simulink model "I_for_8_coils_diagonal_motion"  (R2021b)
settings: Solver=FixedStepAuto  StartTime=4400e-6  StopTime=14760e-6  FixedStep=50e-6  RelTol=1e-3
libraries: simulink x12
(part 1 of 6)
settings Model: Creator=teja  LastModifiedBy=teja

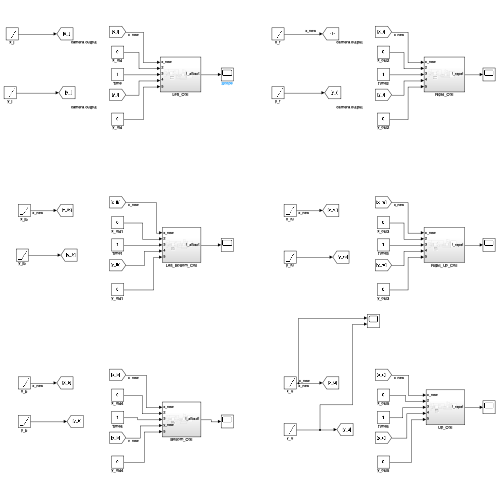
[thumbnail: Simulink's stored preview of the top-level diagram]
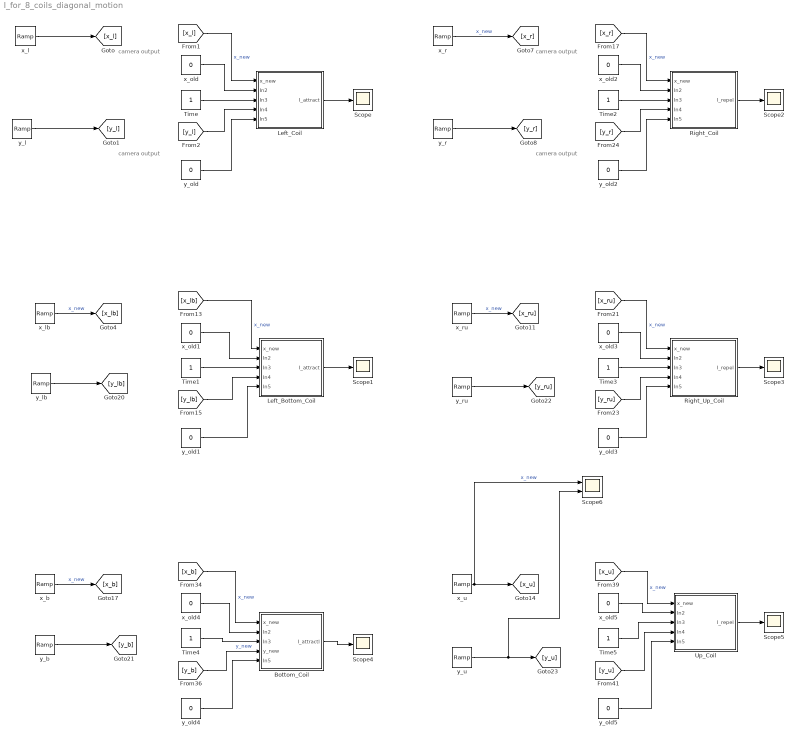
== system I_for_8_coils_diagonal_motion ==
  note: camera output
  note: camera output
  note: camera output
  note: camera output
  Bottom_Coil : Subsystem
  Left_Bottom_Coil : Subsystem
  Left_Coil : Subsystem
  Right_Coil : Subsystem
  Right_Up_Coil : Subsystem
  Scope{,1..5} (6 alike) : Scope
  Scope6 : Scope  NumInputPorts=2
  Time{,1..5} (6 alike) : Constant
  Up_Coil : Subsystem
  x_b : simulink/Sources/Ramp  slope=1  start=0  InitialOutput=-4400e-6
  x_l : simulink/Sources/Ramp  slope=1  start=0  InitialOutput=0
  x_lb : simulink/Sources/Ramp  slope=1  start=0  InitialOutput=0
  x_old{,1..5} (6 alike) : Constant  Value=0
  x_r : simulink/Sources/Ramp  slope=-1  start=0  InitialOutput=-4400e-6
  x_ru : simulink/Sources/Ramp  slope=-1  start=0  InitialOutput=0
  x_u : simulink/Sources/Ramp  slope=-1  start=0  InitialOutput=8800e-6
  y_b : simulink/Sources/Ramp  slope=1  start=0  InitialOutput=0
  y_l : simulink/Sources/Ramp  slope=1  start=0  InitialOutput=-8800e-6
  y_lb : simulink/Sources/Ramp  slope=1  start=0  InitialOutput=0
  y_old{,1..5} (6 alike) : Constant  Value=0
  y_r : simulink/Sources/Ramp  slope=-1  start=4400e-6  InitialOutput=0
  y_ru : simulink/Sources/Ramp  slope=-1  start=0  InitialOutput=0
  y_u : simulink/Sources/Ramp  slope=-1  start=0  InitialOutput=0
  wires:
  y_l/1 -> [y_l]
  x_lb/1 -> [x_lb]  "x_new"
  x_l/1 -> [x_l]
  y_lb/1 -> [y_lb]
  [x_l] -> Left_Coil/1(x_new)  "x_new"
  x_old/1 -> Left_Coil/2(In2)
  Time/1 -> Left_Coil/3(In3)
  [y_l] -> Left_Coil/4(In4)
  y_old/1 -> Left_Coil/5(In5)
  Left_Coil/1(I_attract) -> Scope/1
  [x_lb] -> Left_Bottom_Coil/1(x_new)  "x_new"
  x_old1/1 -> Left_Bottom_Coil/2(In2)
  Time1/1 -> Left_Bottom_Coil/3(In3)
  [y_lb] -> Left_Bottom_Coil/4(In4)
  y_old1/1 -> Left_Bottom_Coil/5(In5)
  Left_Bottom_Coil/1(I_attract) -> Scope1/1
  [x_b] -> Bottom_Coil/1(x_new)  "x_new"
  x_old4/1 -> Bottom_Coil/2(In2)
  Time4/1 -> Bottom_Coil/3(In3)
  [y_b] -> Bottom_Coil/4(y_new)  "y_new"
  y_old4/1 -> Bottom_Coil/5(In5)
  Bottom_Coil/1(I_attractl) -> Scope4/1
  [x_r] -> Right_Coil/1(x_new)  "x_new"
  x_old2/1 -> Right_Coil/2(In2)
  Time2/1 -> Right_Coil/3(In3)
  [y_r] -> Right_Coil/4(In4)
  y_old2/1 -> Right_Coil/5(In5)
  Right_Coil/1(I_repel) -> Scope2/1
  [x_ru] -> Right_Up_Coil/1(x_new)  "x_new"
  x_old3/1 -> Right_Up_Coil/2(In2)
  Time3/1 -> Right_Up_Coil/3(In3)
  [y_ru] -> Right_Up_Coil/4(In4)
  y_old3/1 -> Right_Up_Coil/5(In5)
  Right_Up_Coil/1(I_repel) -> Scope3/1
  [x_u] -> Up_Coil/1(x_new)  "x_new"
  x_old5/1 -> Up_Coil/2(In2)
  Time5/1 -> Up_Coil/3(In3)
  [y_u] -> Up_Coil/4(In4)
  y_old5/1 -> Up_Coil/5(In5)
  Up_Coil/1(I_repel) -> Scope5/1
  y_b/1 -> [y_b]
  x_b/1 -> [x_b]  "x_new"
  x_r/1 -> [x_r]  "x_new"
  y_r/1 -> [y_r]
  y_ru/1 -> [y_ru]
  x_ru/1 -> [x_ru]  "x_new"
  y_u/1 -> Scope6/2, [y_u]
  x_u/1 -> Scope6/1, [x_u]  "x_new"

== system I_for_8_coils_diagonal_motion/Bottom_Coil ==
  note: Inside coil, it is repulsive force, hence outside coil it generates attractive force
      |
      | Hence F increasing from -14 to -4
  note: Bot coming to this coil
  x_new : Inport
  In2 : Inport  Port=2
  In3 : Inport  Port=3
  y_new : Inport  Port=4
  In5 : Inport  Port=5
  Force_repel2 : Subsystem
  Left_Coil2 : Subsystem
  Required Current in Coil4 : MATLAB Function  TreatAsAtomicUnit=on
  z_new4 : Constant  Value=150e-6
  I_attractl : Outport
  wires:
  In2/1 -> Force_repel2/2(In2)
  In3/1 -> Force_repel2/3(In3)
  In5/1 -> Force_repel2/5(In5)
  x_new/1 -> Left_Coil2/1(x_new), Required Current in Coil4/7(x_new), Force_repel2/1(In1)
  Required Current in Coil4/1(I) -> I_attractl/1  "I_attract"
  Left_Coil2/4(Out4) -> Required Current in Coil4/6(dyn_dz)  "dyn/dz"
  y_new/1 -> Left_Coil2/2(y_new), Required Current in Coil4/8(y_new), Force_repel2/4(In4)
  Force_repel2/1(F_mag_x) -> [F_mag_xb]  "F_mag_x"
  z_new4/1 -> Left_Coil2/3(z_new)
  [F_mag_xb] -> Required Current in Coil4/1(F_xz_1)  "F_x"
  [F_mag_yb] -> Required Current in Coil4/2(F_yz_1)  "F_y"
  Force_repel2/2(F_mag_y) -> [F_mag_yb]
  Left_Coil2/2(Out2) -> Required Current in Coil4/4(dxn_dz)  "dxn/dz"
  Left_Coil2/1(Out1) -> Required Current in Coil4/3(dxp_dz)  "dxp/dz"
  Left_Coil2/3(Out3) -> Required Current in Coil4/5(dyp_dz)  "dyp/dz"

== system I_for_8_coils_diagonal_motion/Left_Bottom_Coil ==
  note: Inside coil, it is repulsive force, hence outside coil it generates attractive force
      |
      | Hence F increasing from -14 to -4
  note: Bot coming to this coil
  x_new : Inport
  In2 : Inport  Port=2
  In3 : Inport  Port=3
  In4 : Inport  Port=4
  In5 : Inport  Port=5
  Force_repel : Subsystem
  Left_Coil : Subsystem
  Required Current in Coil1 : MATLAB Function  TreatAsAtomicUnit=on
  z_new1 : Constant  Value=150e-6
  I_attract : Outport
  wires:
  In3/1 -> Force_repel/3(In3)
  In2/1 -> Force_repel/2(In2)
  x_new/1 -> Required Current in Coil1/7(x_new), Left_Coil/1(x_new), Force_repel/1(In1)
  [F_mag_ylb] -> Required Current in Coil1/2(F_yz_1)  "F_y"
  Force_repel/2(F_mag_y) -> [F_mag_ylb]
  Left_Coil/4(Out4) -> Required Current in Coil1/6(dyn_dz)  "dyn/dz"
  Force_repel/1(F_mag_x) -> [F_mag_xlb]  "F_mag_x"
  In5/1 -> Force_repel/5(In5)
  Required Current in Coil1/1(I) -> I_attract/1  "I_attract"
  [F_mag_xlb] -> Required Current in Coil1/1(F_xz_1)  "F_x"
  Left_Coil/1(Out1) -> Required Current in Coil1/3(dxp_dz)  "dxp/dz"
  In4/1 -> Required Current in Coil1/8(y_new), Left_Coil/2(y_new), Force_repel/4(In4)
  z_new1/1 -> Left_Coil/3(z_new)
  Left_Coil/2(Out2) -> Required Current in Coil1/4(dxn_dz)  "dxn/dz"
  Left_Coil/3(Out3) -> Required Current in Coil1/5(dyp_dz)  "dyp/dz"

== system I_for_8_coils_diagonal_motion/Left_Coil ==
  note: Inside coil, it is attractive force, hence outside coil it generates repulsive force
      |
      | Hence F increasing from 4 to 14
  x_new : Inport
  In2 : Inport  Port=2
  In3 : Inport  Port=3
  In4 : Inport  Port=4
  In5 : Inport  Port=5
  Force_attract : Subsystem
  Required Current in Coil : MATLAB Function  TreatAsAtomicUnit=on
  Right_Coil : Subsystem
  z_new : Constant  Value=150e-6
  I_attract : Outport
  wires:
  In2/1 -> Force_attract/2(In2)
  Required Current in Coil/1(I) -> I_attract/1  "I_attract"
  In4/1 -> Right_Coil/2(y_new), Required Current in Coil/8(y_new), Force_attract/4(In4)
  x_new/1 -> Right_Coil/1(x_new), Required Current in Coil/7(x_new), Force_attract/1(In1)
  In3/1 -> Force_attract/3(In3)
  Force_attract/2(F_mag_y) -> [F_mag_yl]
  Right_Coil/1(Out1) -> Required Current in Coil/3(dxp_dz)  "dxp/dz"
  In5/1 -> Force_attract/5(In5)
  z_new/1 -> Right_Coil/3(z_new)
  Right_Coil/2(Out2) -> Required Current in Coil/4(dxn_dz)  "dxn/dz"
  [F_mag_xl] -> Required Current in Coil/1(F_xz_1)  "F_x"
  [F_mag_yl] -> Required Current in Coil/2(F_yz_1)  "F_y"
  Right_Coil/3(Out3) -> Required Current in Coil/5(dyp_dz)  "dyp/dz"
  Force_attract/1(F_mag_x) -> [F_mag_xl]  "F_mag_l"
  Right_Coil/4(Out4) -> Required Current in Coil/6(dyn_dz)  "dyn/dz"

== system I_for_8_coils_diagonal_motion/Right_Coil ==
  note: Bot going away from this coil
  note: Inside coil, it is attractive force, hence outside coil it generates repulsive force
      |
      | Hence F increasing from 4 to 14
  x_new : Inport
  In2 : Inport  Port=2
  In3 : Inport  Port=3
  In4 : Inport  Port=4
  In5 : Inport  Port=5
  Force_attract1 : Subsystem
  Required Current in Coil2 : MATLAB Function  TreatAsAtomicUnit=on
  Right_Coil1 : Subsystem
  z_new2 : Constant  Value=150e-6
  I_repel : Outport
  wires:
  In5/1 -> Force_attract1/5(In5)
  In2/1 -> Force_attract1/2(In2)
  Right_Coil1/1(Out1) -> Required Current in Coil2/3(dxp_dz)  "dxp/dz"
  x_new/1 -> Required Current in Coil2/7(x_new), Right_Coil1/1(x_new), Force_attract1/1(In1)
  Right_Coil1/2(Out2) -> Required Current in Coil2/4(dxn_dz)  "dxn/dz"
  [F_mag_yr] -> Required Current in Coil2/2(F_yz_1)  "F_y"
  In4/1 -> Required Current in Coil2/8(y_new), Right_Coil1/2(y_new), Force_attract1/4(In4)
  z_new2/1 -> Right_Coil1/3(z_new)
  Right_Coil1/3(Out3) -> Required Current in Coil2/5(dyp_dz)  "dyp/dz"
  Force_attract1/1(F_mag_x) -> [F_mag_xr]  "F_mag_x"
  Required Current in Coil2/1(I) -> I_repel/1  "I_repel"
  Force_attract1/2(F_mag_y) -> [F_mag_yr]
  In3/1 -> Force_attract1/3(In3)
  Right_Coil1/4(Out4) -> Required Current in Coil2/6(dyn_dz)  "dyn/dz"
  [F_mag_xr] -> Required Current in Coil2/1(F_xz_1)  "F_x"

== system I_for_8_coils_diagonal_motion/Right_Up_Coil ==
  note: Inside coil, it is repulsive force, hence outside coil it generates attractive force
      |
      | Hence F increasing from -14 to -4
  x_new : Inport
  In2 : Inport  Port=2
  In3 : Inport  Port=3
  In4 : Inport  Port=4
  In5 : Inport  Port=5
  Force_repel1 : Subsystem
  Left_Coil1 : Subsystem
  Required Current in Coil3 : MATLAB Function  TreatAsAtomicUnit=on
  z_new3 : Constant  Value=150e-6
  I_repel : Outport
  wires:
  In2/1 -> Force_repel1/2(In2)
  In3/1 -> Force_repel1/3(In3)
  Left_Coil1/1(Out1) -> Required Current in Coil3/3(dxp_dz)  "dxp/dz"
  In4/1 -> Required Current in Coil3/8(y_new), Left_Coil1/2(y_new), Force_repel1/4(In4)
  z_new3/1 -> Left_Coil1/3(z_new)
  Left_Coil1/3(Out3) -> Required Current in Coil3/5(dyp_dz)  "dyp/dz"
  [F_mag_xru] -> Required Current in Coil3/1(F_xz_1)  "F_x"
  Force_repel1/2(F_mag_y) -> [F_mag_yru]
  Required Current in Coil3/1(I) -> I_repel/1  "I_repel"
  x_new/1 -> Required Current in Coil3/7(x_new), Left_Coil1/1(x_new), Force_repel1/1(In1)
  In5/1 -> Force_repel1/5(In5)
  Left_Coil1/2(Out2) -> Required Current in Coil3/4(dxn_dz)  "dxn/dz"
  Left_Coil1/4(Out4) -> Required Current in Coil3/6(dyn_dz)  "dyn/dz"
  [F_mag_yru] -> Required Current in Coil3/2(F_yz_1)  "F_y"
  Force_repel1/1(F_mag_x) -> [F_mag_xru]  "F_mag_x"

== system I_for_8_coils_diagonal_motion/Up_Coil ==
  note: Inside coil, it is repulsive force, hence outside coil it generates attractive force
      |
      | Hence F increasing from -14 to -4
  note: Bot coming to this coil
  x_new : Inport
  In2 : Inport  Port=2
  In3 : Inport  Port=3
  In4 : Inport  Port=4
  In5 : Inport  Port=5
  Force_repel3 : Subsystem
  Left_Coil3 : Subsystem
  Required Current in Coil5 : MATLAB Function  TreatAsAtomicUnit=on
  z_new5 : Constant  Value=150e-6
  I_repel : Outport
  wires:
  In2/1 -> Force_repel3/2(In2)
  In5/1 -> Force_repel3/5(In5)
  Required Current in Coil5/1(I) -> I_repel/1  "I_repel"
  Force_repel3/2(F_mag_y) -> [F_mag_yu]
  [F_mag_xu] -> Required Current in Coil5/1(F_xz_1)  "F_x"
  [F_mag_yu] -> Required Current in Coil5/2(F_yz_1)  "F_y"
  In4/1 -> Required Current in Coil5/8(y_new), Left_Coil3/2(y_new), Force_repel3/4(In4)
  z_new5/1 -> Left_Coil3/3(z_new)
  In3/1 -> Force_repel3/3(In3)
  x_new/1 -> Required Current in Coil5/7(x_new), Left_Coil3/1(x_new), Force_repel3/1(In1)
  Force_repel3/1(F_mag_x) -> [F_mag_xu]  "F_mag_x"
  Left_Coil3/2(Out2) -> Required Current in Coil5/4(dxn_dz)  "dxn/dz"
  Left_Coil3/3(Out3) -> Required Current in Coil5/5(dyp_dz)  "dyp/dz"
  Left_Coil3/1(Out1) -> Required Current in Coil5/3(dxp_dz)  "dxp/dz"
  Left_Coil3/4(Out4) -> Required Current in Coil5/6(dyn_dz)  "dyn/dz"

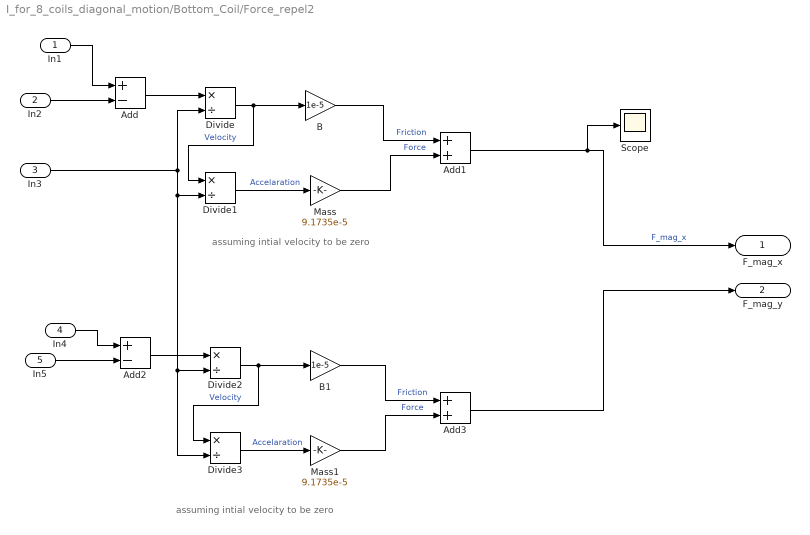
== system I_for_8_coils_diagonal_motion/Bottom_Coil/Force_repel2 ==
  note: assuming intial velocity to be zero
  note: assuming intial velocity to be zero
  In1 : Inport
  In2 : Inport  Port=2
  In3 : Inport  Port=3
  In4 : Inport  Port=4
  In5 : Inport  Port=5
  Add : Sum  Inputs=+-
  Add1 : Sum
  Add2 : Sum  Inputs=+-
  Add3 : Sum
  B : Gain  Gain=1e-5
  B1 : Gain  Gain=1e-5
  Divide{,1..3} (4 alike) : Product  Inputs=*/
  Mass : Gain  Gain=9.1735e-5
  Mass1 : Gain  Gain=9.1735e-5
  Scope : Scope
  F_mag_x : Outport
  F_mag_y : Outport  Port=2
  wires:
  Add3/1 -> F_mag_y/1
  In4/1 -> Add2/1
  In5/1 -> Add2/2
  Mass/1 -> Add1/2  "Force"
  Add2/1 -> Divide2/1
  B1/1 -> Add3/1  "Friction"
  Mass1/1 -> Add3/2  "Force"
  B/1 -> Add1/1  "Friction"
  In1/1 -> Add/1
  Divide/1 -> Divide1/1, B/1  "Velocity"
  Add/1 -> Divide/1
  Divide2/1 -> B1/1, Divide3/1  "Velocity"
  Divide3/1 -> Mass1/1  "Accelaration"
  Divide1/1 -> Mass/1  "Accelaration"
  In3/1 -> Divide3/2, Divide2/2, Divide1/2, Divide/2
  In2/1 -> Add/2
  Add1/1 -> Scope/1, F_mag_x/1  "F_mag_x"

== system I_for_8_coils_diagonal_motion/Bottom_Coil/Left_Coil2 ==
  x_new : Inport
  y_new : Inport  Port=2
  z_new : Inport  Port=3
  Add{,1..3} (4 alike) : Sum
  Inner 5 Coils : Subsystem
  Outer5 Coils : Subsystem
  Out1 : Outport
  Out2 : Outport  Port=2
  Out3 : Outport  Port=3
  Out4 : Outport  Port=4
  wires:
  Add2/1 -> Out3/1
  Add1/1 -> Out2/1
  Outer5 Coils/2(Out2) -> Add1/2
  Outer5 Coils/3(Out3) -> Add2/2
  Add/1 -> Out1/1
  Inner 5 Coils/3(Out3) -> Add2/1
  Add3/1 -> Out4/1
  Inner 5 Coils/4(Out4) -> Add3/1
  x_new/1 -> Outer5 Coils/1(x_new), Inner 5 Coils/1(x_new)
  Inner 5 Coils/2(Out2) -> Add1/1
  Inner 5 Coils/1(Out1) -> Add/1
  y_new/1 -> Outer5 Coils/2(y_new), Inner 5 Coils/2(y_new)
  Outer5 Coils/1(Out1) -> Add/2
  Outer5 Coils/4(Out4) -> Add3/2
  z_new/1 -> Outer5 Coils/3(z_new), Inner 5 Coils/3(z_new)

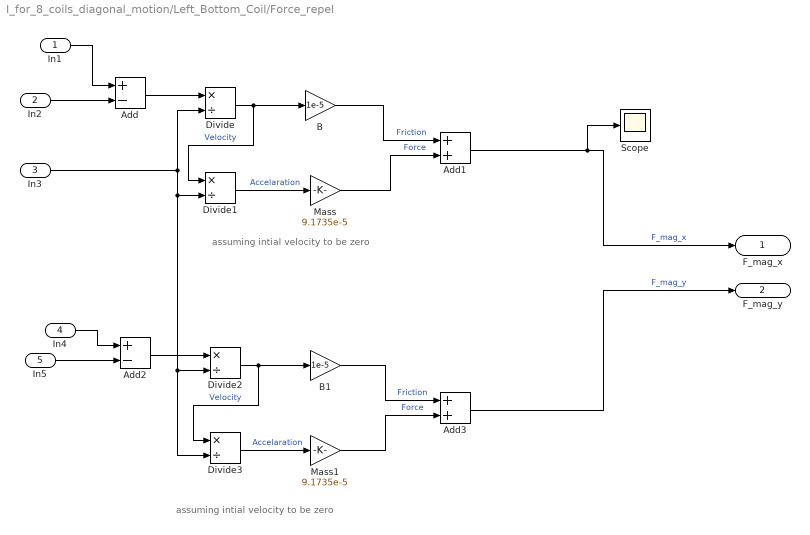
== system I_for_8_coils_diagonal_motion/Left_Bottom_Coil/Force_repel ==
  note: assuming intial velocity to be zero
  note: assuming intial velocity to be zero
  In1 : Inport
  In2 : Inport  Port=2
  In3 : Inport  Port=3
  In4 : Inport  Port=4
  In5 : Inport  Port=5
  Add : Sum  Inputs=+-
  Add1 : Sum
  Add2 : Sum  Inputs=+-
  Add3 : Sum
  B : Gain  Gain=1e-5
  B1 : Gain  Gain=1e-5
  Divide{,1..3} (4 alike) : Product  Inputs=*/
  Mass : Gain  Gain=9.1735e-5
  Mass1 : Gain  Gain=9.1735e-5
  Scope : Scope
  F_mag_x : Outport
  F_mag_y : Outport  Port=2
  wires:
  Add1/1 -> F_mag_x/1, Scope/1  "F_mag_x"
  In2/1 -> Add/2
  In3/1 -> Divide/2, Divide1/2, Divide2/2, Divide3/2
  Divide1/1 -> Mass/1  "Accelaration"
  Divide3/1 -> Mass1/1  "Accelaration"
  Divide2/1 -> Divide3/1, B1/1  "Velocity"
  Add/1 -> Divide/1
  Divide/1 -> B/1, Divide1/1  "Velocity"
  In1/1 -> Add/1
  B/1 -> Add1/1  "Friction"
  Mass1/1 -> Add3/2  "Force"
  B1/1 -> Add3/1  "Friction"
  Add2/1 -> Divide2/1
  Mass/1 -> Add1/2  "Force"
  In5/1 -> Add2/2
  Add3/1 -> F_mag_y/1  "F_mag_y"
  In4/1 -> Add2/1

== system I_for_8_coils_diagonal_motion/Left_Bottom_Coil/Left_Coil ==
  x_new : Inport
  y_new : Inport  Port=2
  z_new : Inport  Port=3
  Add{,1..3} (4 alike) : Sum
  Inner 5 Coils : Subsystem
  Outer5 Coils : Subsystem
  Out1 : Outport
  Out2 : Outport  Port=2
  Out3 : Outport  Port=3
  Out4 : Outport  Port=4
  wires:
  z_new/1 -> Inner 5 Coils/3(z_new), Outer5 Coils/3(z_new)
  Outer5 Coils/4(Out4) -> Add3/2
  Outer5 Coils/1(Out1) -> Add/2
  y_new/1 -> Inner 5 Coils/2(y_new), Outer5 Coils/2(y_new)
  Inner 5 Coils/1(Out1) -> Add/1
  Inner 5 Coils/2(Out2) -> Add1/1
  x_new/1 -> Inner 5 Coils/1(x_new), Outer5 Coils/1(x_new)
  Inner 5 Coils/4(Out4) -> Add3/1
  Add3/1 -> Out4/1
  Inner 5 Coils/3(Out3) -> Add2/1
  Add/1 -> Out1/1
  Outer5 Coils/3(Out3) -> Add2/2
  Outer5 Coils/2(Out2) -> Add1/2
  Add1/1 -> Out2/1
  Add2/1 -> Out3/1

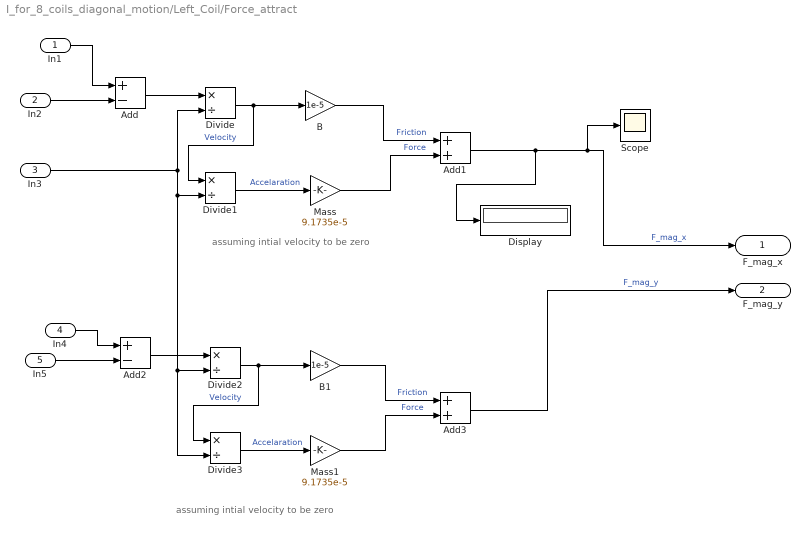
== system I_for_8_coils_diagonal_motion/Left_Coil/Force_attract ==
  note: assuming intial velocity to be zero
  note: assuming intial velocity to be zero
  In1 : Inport
  In2 : Inport  Port=2
  In3 : Inport  Port=3
  In4 : Inport  Port=4
  In5 : Inport  Port=5
  Add : Sum  Inputs=+-
  Add1 : Sum
  Add2 : Sum  Inputs=+-
  Add3 : Sum
  B : Gain  Gain=1e-5
  B1 : Gain  Gain=1e-5
  Display : Display
  Divide{,1..3} (4 alike) : Product  Inputs=*/
  Mass : Gain  Gain=9.1735e-5
  Mass1 : Gain  Gain=9.1735e-5
  Scope : Scope
  F_mag_x : Outport
  F_mag_y : Outport  Port=2
  wires:
  In4/1 -> Add2/1
  Add3/1 -> F_mag_y/1  "F_mag_y"
  In5/1 -> Add2/2
  Mass/1 -> Add1/2  "Force"
  Add2/1 -> Divide2/1
  B1/1 -> Add3/1  "Friction"
  Mass1/1 -> Add3/2  "Force"
  B/1 -> Add1/1  "Friction"
  In1/1 -> Add/1
  Divide/1 -> Divide1/1, B/1  "Velocity"
  Add/1 -> Divide/1
  Divide2/1 -> B1/1, Divide3/1  "Velocity"
  Divide3/1 -> Mass1/1  "Accelaration"
  Divide1/1 -> Mass/1  "Accelaration"
  In3/1 -> Divide3/2, Divide2/2, Divide1/2, Divide/2
  In2/1 -> Add/2
  Add1/1 -> Display/1, Scope/1, F_mag_x/1  "F_mag_x"

== system I_for_8_coils_diagonal_motion/Left_Coil/Right_Coil ==
  x_new : Inport
  y_new : Inport  Port=2
  z_new : Inport  Port=3
  Add{,1..3} (4 alike) : Sum
  Inner 5 Coils : Subsystem
  Outer5 Coils : Subsystem
  Out1 : Outport
  Out2 : Outport  Port=2
  Out3 : Outport  Port=3
  Out4 : Outport  Port=4
  wires:
  Add2/1 -> Out3/1
  Add1/1 -> Out2/1
  Outer5 Coils/2(Out2) -> Add1/2
  Outer5 Coils/3(Out3) -> Add2/2
  Add/1 -> Out1/1
  Inner 5 Coils/3(Out3) -> Add2/1
  Add3/1 -> Out4/1
  Inner 5 Coils/4(Out4) -> Add3/1
  x_new/1 -> Outer5 Coils/1(x_new), Inner 5 Coils/1(x_new)
  Inner 5 Coils/2(Out2) -> Add1/1
  Inner 5 Coils/1(Out1) -> Add/1
  y_new/1 -> Outer5 Coils/2(y_new), Inner 5 Coils/2(y_new)
  Outer5 Coils/1(Out1) -> Add/2
  Outer5 Coils/4(Out4) -> Add3/2
  z_new/1 -> Outer5 Coils/3(z_new), Inner 5 Coils/3(z_new)

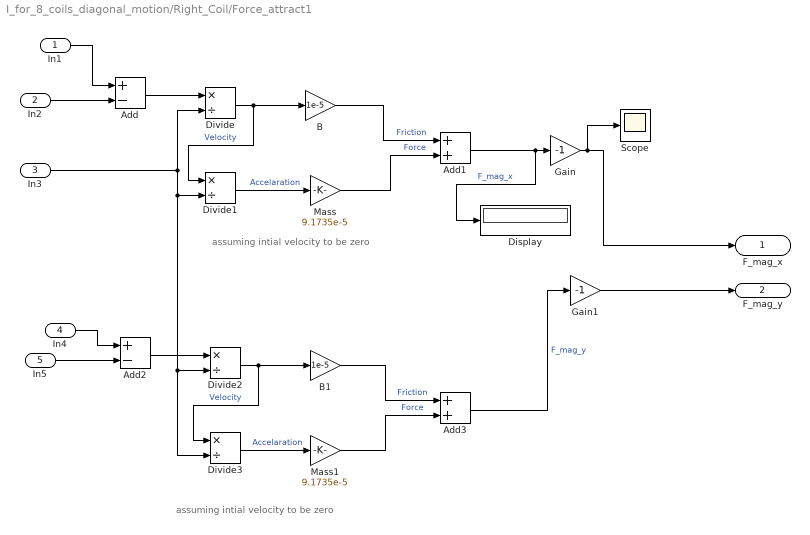
== system I_for_8_coils_diagonal_motion/Right_Coil/Force_attract1 ==
  note: assuming intial velocity to be zero
  note: assuming intial velocity to be zero
  In1 : Inport
  In2 : Inport  Port=2
  In3 : Inport  Port=3
  In4 : Inport  Port=4
  In5 : Inport  Port=5
  Add : Sum  Inputs=+-
  Add1 : Sum
  Add2 : Sum  Inputs=+-
  Add3 : Sum
  B : Gain  Gain=1e-5
  B1 : Gain  Gain=1e-5
  Display : Display
  Divide{,1..3} (4 alike) : Product  Inputs=*/
  Gain : Gain  Gain=-1
  Gain1 : Gain  Gain=-1
  Mass : Gain  Gain=9.1735e-5
  Mass1 : Gain  Gain=9.1735e-5
  Scope : Scope
  F_mag_x : Outport
  F_mag_y : Outport  Port=2
  wires:
  Add1/1 -> Gain/1, Display/1  "F_mag_x"
  In2/1 -> Add/2
  In3/1 -> Divide/2, Divide1/2, Divide2/2, Divide3/2
  Divide1/1 -> Mass/1  "Accelaration"
  Divide3/1 -> Mass1/1  "Accelaration"
  Divide2/1 -> Divide3/1, B1/1  "Velocity"
  Add/1 -> Divide/1
  Divide/1 -> B/1, Divide1/1  "Velocity"
  In1/1 -> Add/1
  B/1 -> Add1/1  "Friction"
  Mass1/1 -> Add3/2  "Force"
  B1/1 -> Add3/1  "Friction"
  Add2/1 -> Divide2/1
  Mass/1 -> Add1/2  "Force"
  In5/1 -> Add2/2
  Add3/1 -> Gain1/1  "F_mag_y"
  In4/1 -> Add2/1
  Gain/1 -> F_mag_x/1, Scope/1
  Gain1/1 -> F_mag_y/1

== system I_for_8_coils_diagonal_motion/Right_Coil/Right_Coil1 ==
  x_new : Inport
  y_new : Inport  Port=2
  z_new : Inport  Port=3
  Add{,1..3} (4 alike) : Sum
  Inner 5 Coils : Subsystem
  Outer5 Coils : Subsystem
  Out1 : Outport
  Out2 : Outport  Port=2
  Out3 : Outport  Port=3
  Out4 : Outport  Port=4
  wires:
  z_new/1 -> Inner 5 Coils/3(z_new), Outer5 Coils/3(z_new)
  Outer5 Coils/4(Out4) -> Add3/2
  Outer5 Coils/1(Out1) -> Add/2
  y_new/1 -> Inner 5 Coils/2(y_new), Outer5 Coils/2(y_new)
  Inner 5 Coils/1(Out1) -> Add/1
  Inner 5 Coils/2(Out2) -> Add1/1
  x_new/1 -> Inner 5 Coils/1(x_new), Outer5 Coils/1(x_new)
  Inner 5 Coils/4(Out4) -> Add3/1
  Add3/1 -> Out4/1
  Inner 5 Coils/3(Out3) -> Add2/1
  Add/1 -> Out1/1
  Outer5 Coils/3(Out3) -> Add2/2
  Outer5 Coils/2(Out2) -> Add1/2
  Add1/1 -> Out2/1
  Add2/1 -> Out3/1

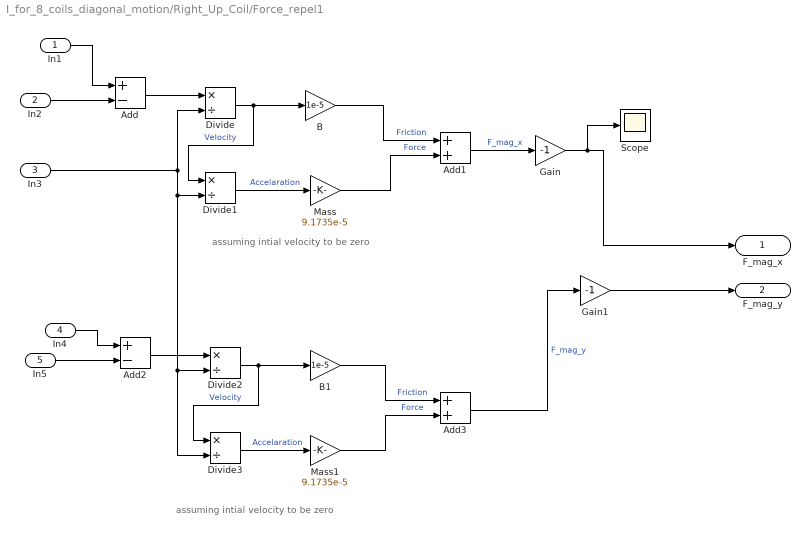
== system I_for_8_coils_diagonal_motion/Right_Up_Coil/Force_repel1 ==
  note: assuming intial velocity to be zero
  note: assuming intial velocity to be zero
  In1 : Inport
  In2 : Inport  Port=2
  In3 : Inport  Port=3
  In4 : Inport  Port=4
  In5 : Inport  Port=5
  Add : Sum  Inputs=+-
  Add1 : Sum
  Add2 : Sum  Inputs=+-
  Add3 : Sum
  B : Gain  Gain=1e-5
  B1 : Gain  Gain=1e-5
  Divide{,1..3} (4 alike) : Product  Inputs=*/
  Gain : Gain  Gain=-1
  Gain1 : Gain  Gain=-1
  Mass : Gain  Gain=9.1735e-5
  Mass1 : Gain  Gain=9.1735e-5
  Scope : Scope
  F_mag_x : Outport
  F_mag_y : Outport  Port=2
  wires:
  Gain1/1 -> F_mag_y/1
  Gain/1 -> Scope/1, F_mag_x/1
  In4/1 -> Add2/1
  Add3/1 -> Gain1/1  "F_mag_y"
  In5/1 -> Add2/2
  Mass/1 -> Add1/2  "Force"
  Add2/1 -> Divide2/1
  B1/1 -> Add3/1  "Friction"
  Mass1/1 -> Add3/2  "Force"
  B/1 -> Add1/1  "Friction"
  In1/1 -> Add/1
  Divide/1 -> Divide1/1, B/1  "Velocity"
  Add/1 -> Divide/1
  Divide2/1 -> B1/1, Divide3/1  "Velocity"
  Divide3/1 -> Mass1/1  "Accelaration"
  Divide1/1 -> Mass/1  "Accelaration"
  In3/1 -> Divide3/2, Divide2/2, Divide1/2, Divide/2
  In2/1 -> Add/2
  Add1/1 -> Gain/1  "F_mag_x"

== system I_for_8_coils_diagonal_motion/Right_Up_Coil/Left_Coil1 ==
  x_new : Inport
  y_new : Inport  Port=2
  z_new : Inport  Port=3
  Add{,1..3} (4 alike) : Sum
  Inner 5 Coils : Subsystem
  Outer5 Coils : Subsystem
  Out1 : Outport
  Out2 : Outport  Port=2
  Out3 : Outport  Port=3
  Out4 : Outport  Port=4
  wires:
  Add2/1 -> Out3/1
  Add1/1 -> Out2/1
  Outer5 Coils/2(Out2) -> Add1/2
  Outer5 Coils/3(Out3) -> Add2/2
  Add/1 -> Out1/1
  Inner 5 Coils/3(Out3) -> Add2/1
  Add3/1 -> Out4/1
  Inner 5 Coils/4(Out4) -> Add3/1
  x_new/1 -> Outer5 Coils/1(x_new), Inner 5 Coils/1(x_new)
  Inner 5 Coils/2(Out2) -> Add1/1
  Inner 5 Coils/1(Out1) -> Add/1
  y_new/1 -> Outer5 Coils/2(y_new), Inner 5 Coils/2(y_new)
  Outer5 Coils/1(Out1) -> Add/2
  Outer5 Coils/4(Out4) -> Add3/2
  z_new/1 -> Outer5 Coils/3(z_new), Inner 5 Coils/3(z_new)

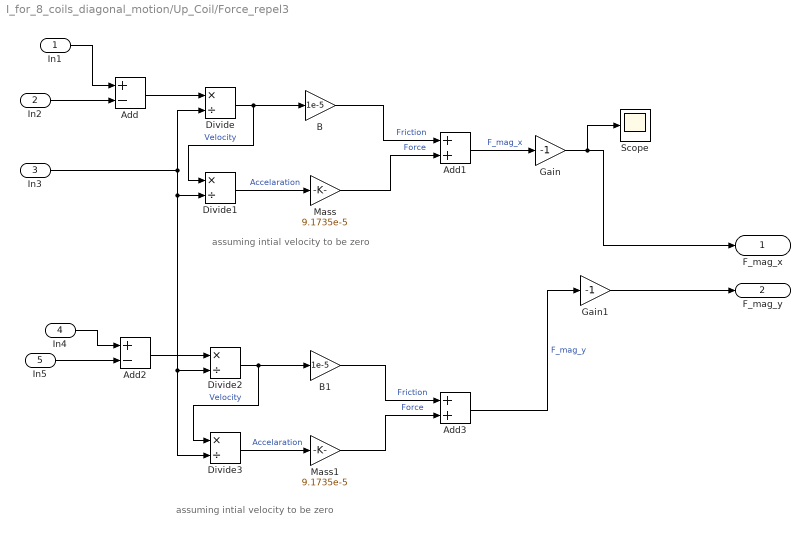
== system I_for_8_coils_diagonal_motion/Up_Coil/Force_repel3 ==
  note: assuming intial velocity to be zero
  note: assuming intial velocity to be zero
  In1 : Inport
  In2 : Inport  Port=2
  In3 : Inport  Port=3
  In4 : Inport  Port=4
  In5 : Inport  Port=5
  Add : Sum  Inputs=+-
  Add1 : Sum
  Add2 : Sum  Inputs=+-
  Add3 : Sum
  B : Gain  Gain=1e-5
  B1 : Gain  Gain=1e-5
  Divide{,1..3} (4 alike) : Product  Inputs=*/
  Gain : Gain  Gain=-1
  Gain1 : Gain  Gain=-1
  Mass : Gain  Gain=9.1735e-5
  Mass1 : Gain  Gain=9.1735e-5
  Scope : Scope
  F_mag_x : Outport
  F_mag_y : Outport  Port=2
  wires:
  Add1/1 -> Gain/1  "F_mag_x"
  In2/1 -> Add/2
  In3/1 -> Divide/2, Divide1/2, Divide2/2, Divide3/2
  Divide1/1 -> Mass/1  "Accelaration"
  Divide3/1 -> Mass1/1  "Accelaration"
  Divide2/1 -> Divide3/1, B1/1  "Velocity"
  Add/1 -> Divide/1
  Divide/1 -> B/1, Divide1/1  "Velocity"
  In1/1 -> Add/1
  B/1 -> Add1/1  "Friction"
  Mass1/1 -> Add3/2  "Force"
  B1/1 -> Add3/1  "Friction"
  Add2/1 -> Divide2/1
  Mass/1 -> Add1/2  "Force"
  In5/1 -> Add2/2
  Add3/1 -> Gain1/1  "F_mag_y"
  In4/1 -> Add2/1
  Gain/1 -> F_mag_x/1, Scope/1
  Gain1/1 -> F_mag_y/1

== system I_for_8_coils_diagonal_motion/Up_Coil/Left_Coil3 ==
  x_new : Inport
  y_new : Inport  Port=2
  z_new : Inport  Port=3
  Add{,1..3} (4 alike) : Sum
  Inner 5 Coils : Subsystem
  Outer5 Coils : Subsystem
  Out1 : Outport
  Out2 : Outport  Port=2
  Out3 : Outport  Port=3
  Out4 : Outport  Port=4
  wires:
  z_new/1 -> Inner 5 Coils/3(z_new), Outer5 Coils/3(z_new)
  Outer5 Coils/4(Out4) -> Add3/2
  Outer5 Coils/1(Out1) -> Add/2
  y_new/1 -> Inner 5 Coils/2(y_new), Outer5 Coils/2(y_new)
  Inner 5 Coils/1(Out1) -> Add/1
  Inner 5 Coils/2(Out2) -> Add1/1
  x_new/1 -> Inner 5 Coils/1(x_new), Outer5 Coils/1(x_new)
  Inner 5 Coils/4(Out4) -> Add3/1
  Add3/1 -> Out4/1
  Inner 5 Coils/3(Out3) -> Add2/1
  Add/1 -> Out1/1
  Outer5 Coils/3(Out3) -> Add2/2
  Outer5 Coils/2(Out2) -> Add1/2
  Add1/1 -> Out2/1
  Add2/1 -> Out3/1

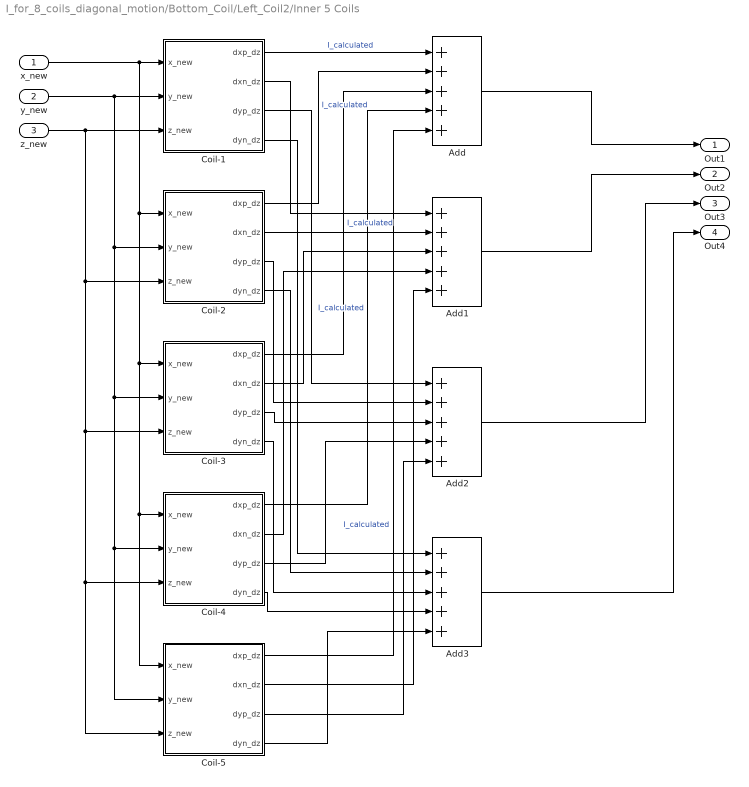
== system I_for_8_coils_diagonal_motion/Bottom_Coil/Left_Coil2/Inner 5 Coils ==
  x_new : Inport
  y_new : Inport  Port=2
  z_new : Inport  Port=3
  Add{,1..3} (4 alike) : Sum  Inputs=+++++
  Coil-1 : MATLAB Function  TreatAsAtomicUnit=on
  Coil-2 : MATLAB Function  TreatAsAtomicUnit=on
  Coil-3 : MATLAB Function  TreatAsAtomicUnit=on
  Coil-4 : MATLAB Function  TreatAsAtomicUnit=on
  Coil-5 : MATLAB Function  TreatAsAtomicUnit=on
  Out1 : Outport
  Out2 : Outport  Port=2
  Out3 : Outport  Port=3
  Out4 : Outport  Port=4
  wires:
  Add2/1 -> Out3/1
  Add1/1 -> Out2/1
  Coil-2/2(dxn_dz) -> Add1/2
  Coil-2/4(dyn_dz) -> Add3/2
  Add3/1 -> Out4/1
  Coil-3/1(dxp_dz) -> Add/3  "I_calculated"
  Coil-3/4(dyn_dz) -> Add3/3
  z_new/1 -> Coil-1/3(z_new), Coil-3/3(z_new), Coil-4/3(z_new), Coil-5/3(z_new), Coil-2/3(z_new)
  Coil-4/1(dxp_dz) -> Add/4  "I_calculated"
  Add/1 -> Out1/1
  Coil-2/1(dxp_dz) -> Add/2  "I_calculated"
  Coil-1/3(dyp_dz) -> Add2/1
  Coil-1/2(dxn_dz) -> Add1/1
  Coil-4/4(dyn_dz) -> Add3/4
  Coil-1/4(dyn_dz) -> Add3/1
  y_new/1 -> Coil-5/2(y_new), Coil-4/2(y_new), Coil-3/2(y_new), Coil-2/2(y_new), Coil-1/2(y_new)
  Coil-5/1(dxp_dz) -> Add/5  "I_calculated"
  x_new/1 -> Coil-5/1(x_new), Coil-4/1(x_new), Coil-3/1(x_new), Coil-2/1(x_new), Coil-1/1(x_new)
  Coil-1/1(dxp_dz) -> Add/1  "I_calculated"
  Coil-2/3(dyp_dz) -> Add2/2
  Coil-5/3(dyp_dz) -> Add2/5
  Coil-4/3(dyp_dz) -> Add2/4
  Coil-5/4(dyn_dz) -> Add3/5
  Coil-4/2(dxn_dz) -> Add1/4
  Coil-3/2(dxn_dz) -> Add1/3
  Coil-3/3(dyp_dz) -> Add2/3
  Coil-5/2(dxn_dz) -> Add1/5

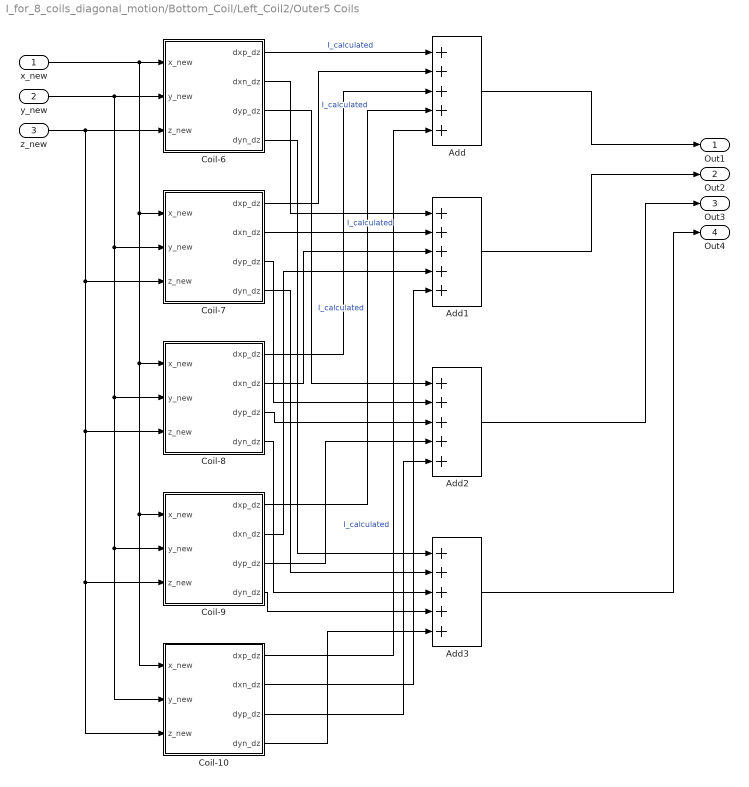
== system I_for_8_coils_diagonal_motion/Bottom_Coil/Left_Coil2/Outer5 Coils ==
  x_new : Inport
  y_new : Inport  Port=2
  z_new : Inport  Port=3
  Add{,1..3} (4 alike) : Sum  Inputs=+++++
  Coil-10 : MATLAB Function  TreatAsAtomicUnit=on
  Coil-6 : MATLAB Function  TreatAsAtomicUnit=on
  Coil-7 : MATLAB Function  TreatAsAtomicUnit=on
  Coil-8 : MATLAB Function  TreatAsAtomicUnit=on
  Coil-9 : MATLAB Function  TreatAsAtomicUnit=on
  Out1 : Outport
  Out2 : Outport  Port=2
  Out3 : Outport  Port=3
  Out4 : Outport  Port=4
  wires:
  Coil-10/2(dxn_dz) -> Add1/5
  Coil-8/3(dyp_dz) -> Add2/3
  Coil-8/2(dxn_dz) -> Add1/3
  Coil-9/2(dxn_dz) -> Add1/4
  Coil-10/4(dyn_dz) -> Add3/5
  Coil-9/3(dyp_dz) -> Add2/4
  Coil-10/3(dyp_dz) -> Add2/5
  Coil-7/3(dyp_dz) -> Add2/2
  Coil-6/1(dxp_dz) -> Add/1  "I_calculated"
  x_new/1 -> Coil-6/1(x_new), Coil-7/1(x_new), Coil-8/1(x_new), Coil-9/1(x_new), Coil-10/1(x_new)
  Coil-10/1(dxp_dz) -> Add/5  "I_calculated"
  y_new/1 -> Coil-6/2(y_new), Coil-7/2(y_new), Coil-8/2(y_new), Coil-9/2(y_new), Coil-10/2(y_new)
  Coil-6/4(dyn_dz) -> Add3/1
  Coil-9/4(dyn_dz) -> Add3/4
  Coil-6/2(dxn_dz) -> Add1/1
  Coil-6/3(dyp_dz) -> Add2/1
  Coil-7/1(dxp_dz) -> Add/2  "I_calculated"
  Add/1 -> Out1/1
  Coil-9/1(dxp_dz) -> Add/4  "I_calculated"
  z_new/1 -> Coil-7/3(z_new), Coil-9/3(z_new), Coil-10/3(z_new), Coil-8/3(z_new), Coil-6/3(z_new)
  Coil-8/4(dyn_dz) -> Add3/3
  Coil-8/1(dxp_dz) -> Add/3  "I_calculated"
  Add3/1 -> Out4/1
  Coil-7/4(dyn_dz) -> Add3/2
  Coil-7/2(dxn_dz) -> Add1/2
  Add1/1 -> Out2/1
  Add2/1 -> Out3/1

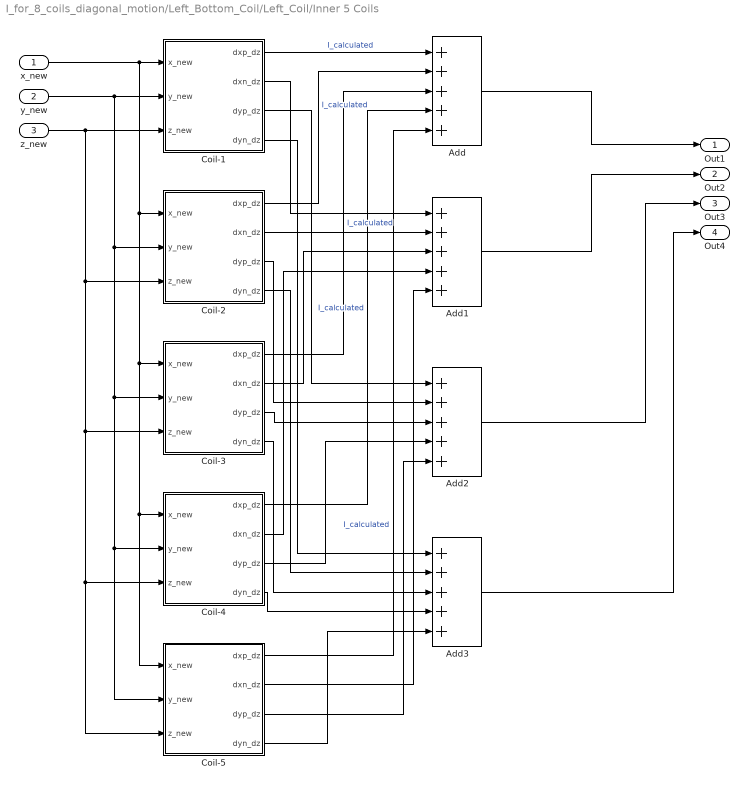
== system I_for_8_coils_diagonal_motion/Left_Bottom_Coil/Left_Coil/Inner 5 Coils ==
  x_new : Inport
  y_new : Inport  Port=2
  z_new : Inport  Port=3
  Add{,1..3} (4 alike) : Sum  Inputs=+++++
  Coil-1 : MATLAB Function  TreatAsAtomicUnit=on
  Coil-2 : MATLAB Function  TreatAsAtomicUnit=on
  Coil-3 : MATLAB Function  TreatAsAtomicUnit=on
  Coil-4 : MATLAB Function  TreatAsAtomicUnit=on
  Coil-5 : MATLAB Function  TreatAsAtomicUnit=on
  Out1 : Outport
  Out2 : Outport  Port=2
  Out3 : Outport  Port=3
  Out4 : Outport  Port=4
  wires:
  Coil-5/2(dxn_dz) -> Add1/5
  Coil-3/3(dyp_dz) -> Add2/3
  Coil-3/2(dxn_dz) -> Add1/3
  Coil-4/2(dxn_dz) -> Add1/4
  Coil-5/4(dyn_dz) -> Add3/5
  Coil-4/3(dyp_dz) -> Add2/4
  Coil-5/3(dyp_dz) -> Add2/5
  Coil-2/3(dyp_dz) -> Add2/2
  Coil-1/1(dxp_dz) -> Add/1  "I_calculated"
  x_new/1 -> Coil-1/1(x_new), Coil-2/1(x_new), Coil-3/1(x_new), Coil-4/1(x_new), Coil-5/1(x_new)
  Coil-5/1(dxp_dz) -> Add/5  "I_calculated"
  y_new/1 -> Coil-1/2(y_new), Coil-2/2(y_new), Coil-3/2(y_new), Coil-4/2(y_new), Coil-5/2(y_new)
  Coil-1/4(dyn_dz) -> Add3/1
  Coil-4/4(dyn_dz) -> Add3/4
  Coil-1/2(dxn_dz) -> Add1/1
  Coil-1/3(dyp_dz) -> Add2/1
  Coil-2/1(dxp_dz) -> Add/2  "I_calculated"
  Add/1 -> Out1/1
  Coil-4/1(dxp_dz) -> Add/4  "I_calculated"
  z_new/1 -> Coil-2/3(z_new), Coil-5/3(z_new), Coil-4/3(z_new), Coil-3/3(z_new), Coil-1/3(z_new)
  Coil-3/4(dyn_dz) -> Add3/3
  Coil-3/1(dxp_dz) -> Add/3  "I_calculated"
  Add3/1 -> Out4/1
  Coil-2/4(dyn_dz) -> Add3/2
  Coil-2/2(dxn_dz) -> Add1/2
  Add1/1 -> Out2/1
  Add2/1 -> Out3/1

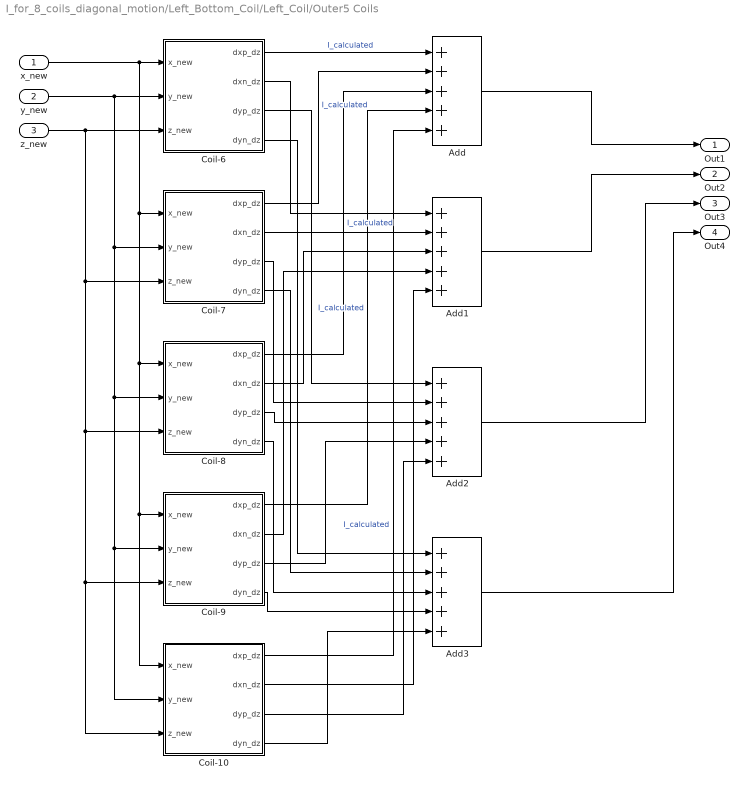
== system I_for_8_coils_diagonal_motion/Left_Bottom_Coil/Left_Coil/Outer5 Coils ==
  x_new : Inport
  y_new : Inport  Port=2
  z_new : Inport  Port=3
  Add{,1..3} (4 alike) : Sum  Inputs=+++++
  Coil-10 : MATLAB Function  TreatAsAtomicUnit=on
  Coil-6 : MATLAB Function  TreatAsAtomicUnit=on
  Coil-7 : MATLAB Function  TreatAsAtomicUnit=on
  Coil-8 : MATLAB Function  TreatAsAtomicUnit=on
  Coil-9 : MATLAB Function  TreatAsAtomicUnit=on
  Out1 : Outport
  Out2 : Outport  Port=2
  Out3 : Outport  Port=3
  Out4 : Outport  Port=4
  wires:
  Add2/1 -> Out3/1
  Add1/1 -> Out2/1
  Coil-7/2(dxn_dz) -> Add1/2
  Coil-7/4(dyn_dz) -> Add3/2
  Add3/1 -> Out4/1
  Coil-8/1(dxp_dz) -> Add/3  "I_calculated"
  Coil-8/4(dyn_dz) -> Add3/3
  z_new/1 -> Coil-6/3(z_new), Coil-8/3(z_new), Coil-10/3(z_new), Coil-9/3(z_new), Coil-7/3(z_new)
  Coil-9/1(dxp_dz) -> Add/4  "I_calculated"
  Add/1 -> Out1/1
  Coil-7/1(dxp_dz) -> Add/2  "I_calculated"
  Coil-6/3(dyp_dz) -> Add2/1
  Coil-6/2(dxn_dz) -> Add1/1
  Coil-9/4(dyn_dz) -> Add3/4
  Coil-6/4(dyn_dz) -> Add3/1
  y_new/1 -> Coil-10/2(y_new), Coil-9/2(y_new), Coil-8/2(y_new), Coil-7/2(y_new), Coil-6/2(y_new)
  Coil-10/1(dxp_dz) -> Add/5  "I_calculated"
  x_new/1 -> Coil-10/1(x_new), Coil-9/1(x_new), Coil-8/1(x_new), Coil-7/1(x_new), Coil-6/1(x_new)
  Coil-6/1(dxp_dz) -> Add/1  "I_calculated"
  Coil-7/3(dyp_dz) -> Add2/2
  Coil-10/3(dyp_dz) -> Add2/5
  Coil-9/3(dyp_dz) -> Add2/4
  Coil-10/4(dyn_dz) -> Add3/5
  Coil-9/2(dxn_dz) -> Add1/4
  Coil-8/2(dxn_dz) -> Add1/3
  Coil-8/3(dyp_dz) -> Add2/3
  Coil-10/2(dxn_dz) -> Add1/5

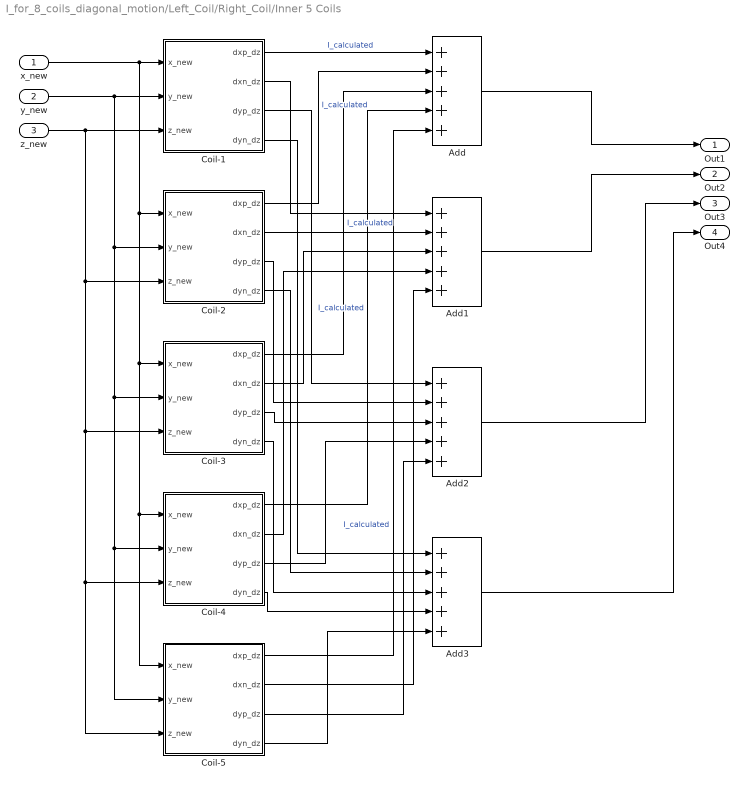
== system I_for_8_coils_diagonal_motion/Left_Coil/Right_Coil/Inner 5 Coils ==
  x_new : Inport
  y_new : Inport  Port=2
  z_new : Inport  Port=3
  Add{,1..3} (4 alike) : Sum  Inputs=+++++
  Coil-1 : MATLAB Function  TreatAsAtomicUnit=on
  Coil-2 : MATLAB Function  TreatAsAtomicUnit=on
  Coil-3 : MATLAB Function  TreatAsAtomicUnit=on
  Coil-4 : MATLAB Function  TreatAsAtomicUnit=on
  Coil-5 : MATLAB Function  TreatAsAtomicUnit=on
  Out1 : Outport
  Out2 : Outport  Port=2
  Out3 : Outport  Port=3
  Out4 : Outport  Port=4
  wires:
  Add2/1 -> Out3/1
  Add1/1 -> Out2/1
  Coil-2/2(dxn_dz) -> Add1/2
  Coil-2/4(dyn_dz) -> Add3/2
  Add3/1 -> Out4/1
  Coil-3/1(dxp_dz) -> Add/3  "I_calculated"
  Coil-3/4(dyn_dz) -> Add3/3
  z_new/1 -> Coil-1/3(z_new), Coil-3/3(z_new), Coil-4/3(z_new), Coil-5/3(z_new), Coil-2/3(z_new)
  Coil-4/1(dxp_dz) -> Add/4  "I_calculated"
  Add/1 -> Out1/1
  Coil-2/1(dxp_dz) -> Add/2  "I_calculated"
  Coil-1/3(dyp_dz) -> Add2/1
  Coil-1/2(dxn_dz) -> Add1/1
  Coil-4/4(dyn_dz) -> Add3/4
  Coil-1/4(dyn_dz) -> Add3/1
  y_new/1 -> Coil-5/2(y_new), Coil-4/2(y_new), Coil-3/2(y_new), Coil-2/2(y_new), Coil-1/2(y_new)
  Coil-5/1(dxp_dz) -> Add/5  "I_calculated"
  x_new/1 -> Coil-5/1(x_new), Coil-4/1(x_new), Coil-3/1(x_new), Coil-2/1(x_new), Coil-1/1(x_new)
  Coil-1/1(dxp_dz) -> Add/1  "I_calculated"
  Coil-2/3(dyp_dz) -> Add2/2
  Coil-5/3(dyp_dz) -> Add2/5
  Coil-4/3(dyp_dz) -> Add2/4
  Coil-5/4(dyn_dz) -> Add3/5
  Coil-4/2(dxn_dz) -> Add1/4
  Coil-3/2(dxn_dz) -> Add1/3
  Coil-3/3(dyp_dz) -> Add2/3
  Coil-5/2(dxn_dz) -> Add1/5

== system I_for_8_coils_diagonal_motion/Left_Coil/Right_Coil/Outer5 Coils ==
  x_new : Inport
  y_new : Inport  Port=2
  z_new : Inport  Port=3
  Add{,1..3} (4 alike) : Sum  Inputs=+++++
  Coil-10 : MATLAB Function  TreatAsAtomicUnit=on
  Coil-6 : MATLAB Function  TreatAsAtomicUnit=on
  Coil-7 : MATLAB Function  TreatAsAtomicUnit=on
  Coil-8 : MATLAB Function  TreatAsAtomicUnit=on
  Coil-9 : MATLAB Function  TreatAsAtomicUnit=on
  Out1 : Outport
  Out2 : Outport  Port=2
  Out3 : Outport  Port=3
  Out4 : Outport  Port=4
  wires:
  Coil-10/2(dxn_dz) -> Add1/5
  Coil-8/3(dyp_dz) -> Add2/3
  Coil-8/2(dxn_dz) -> Add1/3
  Coil-9/2(dxn_dz) -> Add1/4
  Coil-10/4(dyn_dz) -> Add3/5
  Coil-9/3(dyp_dz) -> Add2/4
  Coil-10/3(dyp_dz) -> Add2/5
  Coil-7/3(dyp_dz) -> Add2/2
  Coil-6/1(dxp_dz) -> Add/1  "I_calculated"
  x_new/1 -> Coil-6/1(x_new), Coil-7/1(x_new), Coil-8/1(x_new), Coil-9/1(x_new), Coil-10/1(x_new)
  Coil-10/1(dxp_dz) -> Add/5  "I_calculated"
  y_new/1 -> Coil-6/2(y_new), Coil-7/2(y_new), Coil-8/2(y_new), Coil-9/2(y_new), Coil-10/2(y_new)
  Coil-6/4(dyn_dz) -> Add3/1
  Coil-9/4(dyn_dz) -> Add3/4
  Coil-6/2(dxn_dz) -> Add1/1
  Coil-6/3(dyp_dz) -> Add2/1
  Coil-7/1(dxp_dz) -> Add/2  "I_calculated"
  Add/1 -> Out1/1
  Coil-9/1(dxp_dz) -> Add/4  "I_calculated"
  z_new/1 -> Coil-7/3(z_new), Coil-9/3(z_new), Coil-10/3(z_new), Coil-8/3(z_new), Coil-6/3(z_new)
  Coil-8/4(dyn_dz) -> Add3/3
  Coil-8/1(dxp_dz) -> Add/3  "I_calculated"
  Add3/1 -> Out4/1
  Coil-7/4(dyn_dz) -> Add3/2
  Coil-7/2(dxn_dz) -> Add1/2
  Add1/1 -> Out2/1
  Add2/1 -> Out3/1

== system I_for_8_coils_diagonal_motion/Right_Coil/Right_Coil1/Inner 5 Coils ==
  x_new : Inport
  y_new : Inport  Port=2
  z_new : Inport  Port=3
  Add{,1..3} (4 alike) : Sum  Inputs=+++++
  Coil-1 : MATLAB Function  TreatAsAtomicUnit=on
  Coil-2 : MATLAB Function  TreatAsAtomicUnit=on
  Coil-3 : MATLAB Function  TreatAsAtomicUnit=on
  Coil-4 : MATLAB Function  TreatAsAtomicUnit=on
  Coil-5 : MATLAB Function  TreatAsAtomicUnit=on
  Out1 : Outport
  Out2 : Outport  Port=2
  Out3 : Outport  Port=3
  Out4 : Outport  Port=4
  wires:
  Coil-5/2(dxn_dz) -> Add1/5
  Coil-3/3(dyp_dz) -> Add2/3
  Coil-3/2(dxn_dz) -> Add1/3
  Coil-4/2(dxn_dz) -> Add1/4
  Coil-5/4(dyn_dz) -> Add3/5
  Coil-4/3(dyp_dz) -> Add2/4
  Coil-5/3(dyp_dz) -> Add2/5
  Coil-2/3(dyp_dz) -> Add2/2
  Coil-1/1(dxp_dz) -> Add/1  "I_calculated"
  x_new/1 -> Coil-1/1(x_new), Coil-2/1(x_new), Coil-3/1(x_new), Coil-4/1(x_new), Coil-5/1(x_new)
  Coil-5/1(dxp_dz) -> Add/5  "I_calculated"
  y_new/1 -> Coil-1/2(y_new), Coil-2/2(y_new), Coil-3/2(y_new), Coil-4/2(y_new), Coil-5/2(y_new)
  Coil-1/4(dyn_dz) -> Add3/1
  Coil-4/4(dyn_dz) -> Add3/4
  Coil-1/2(dxn_dz) -> Add1/1
  Coil-1/3(dyp_dz) -> Add2/1
  Coil-2/1(dxp_dz) -> Add/2  "I_calculated"
  Add/1 -> Out1/1
  Coil-4/1(dxp_dz) -> Add/4  "I_calculated"
  z_new/1 -> Coil-2/3(z_new), Coil-5/3(z_new), Coil-4/3(z_new), Coil-3/3(z_new), Coil-1/3(z_new)
  Coil-3/4(dyn_dz) -> Add3/3
  Coil-3/1(dxp_dz) -> Add/3  "I_calculated"
  Add3/1 -> Out4/1
  Coil-2/4(dyn_dz) -> Add3/2
  Coil-2/2(dxn_dz) -> Add1/2
  Add1/1 -> Out2/1
  Add2/1 -> Out3/1

== system I_for_8_coils_diagonal_motion/Right_Coil/Right_Coil1/Outer5 Coils ==
  x_new : Inport
  y_new : Inport  Port=2
  z_new : Inport  Port=3
  Add{,1..3} (4 alike) : Sum  Inputs=+++++
  Coil-10 : MATLAB Function  TreatAsAtomicUnit=on
  Coil-6 : MATLAB Function  TreatAsAtomicUnit=on
  Coil-7 : MATLAB Function  TreatAsAtomicUnit=on
  Coil-8 : MATLAB Function  TreatAsAtomicUnit=on
  Coil-9 : MATLAB Function  TreatAsAtomicUnit=on
  Out1 : Outport
  Out2 : Outport  Port=2
  Out3 : Outport  Port=3
  Out4 : Outport  Port=4
  wires:
  Add2/1 -> Out3/1
  Add1/1 -> Out2/1
  Coil-7/2(dxn_dz) -> Add1/2
  Coil-7/4(dyn_dz) -> Add3/2
  Add3/1 -> Out4/1
  Coil-8/1(dxp_dz) -> Add/3  "I_calculated"
  Coil-8/4(dyn_dz) -> Add3/3
  z_new/1 -> Coil-6/3(z_new), Coil-8/3(z_new), Coil-10/3(z_new), Coil-9/3(z_new), Coil-7/3(z_new)
  Coil-9/1(dxp_dz) -> Add/4  "I_calculated"
  Add/1 -> Out1/1
  Coil-7/1(dxp_dz) -> Add/2  "I_calculated"
  Coil-6/3(dyp_dz) -> Add2/1
  Coil-6/2(dxn_dz) -> Add1/1
  Coil-9/4(dyn_dz) -> Add3/4
  Coil-6/4(dyn_dz) -> Add3/1
  y_new/1 -> Coil-10/2(y_new), Coil-9/2(y_new), Coil-8/2(y_new), Coil-7/2(y_new), Coil-6/2(y_new)
  Coil-10/1(dxp_dz) -> Add/5  "I_calculated"
  x_new/1 -> Coil-10/1(x_new), Coil-9/1(x_new), Coil-8/1(x_new), Coil-7/1(x_new), Coil-6/1(x_new)
  Coil-6/1(dxp_dz) -> Add/1  "I_calculated"
  Coil-7/3(dyp_dz) -> Add2/2
  Coil-10/3(dyp_dz) -> Add2/5
  Coil-9/3(dyp_dz) -> Add2/4
  Coil-10/4(dyn_dz) -> Add3/5
  Coil-9/2(dxn_dz) -> Add1/4
  Coil-8/2(dxn_dz) -> Add1/3
  Coil-8/3(dyp_dz) -> Add2/3
  Coil-10/2(dxn_dz) -> Add1/5

== system I_for_8_coils_diagonal_motion/Right_Up_Coil/Left_Coil1/Inner 5 Coils ==
  x_new : Inport
  y_new : Inport  Port=2
  z_new : Inport  Port=3
  Add{,1..3} (4 alike) : Sum  Inputs=+++++
  Coil-1 : MATLAB Function  TreatAsAtomicUnit=on
  Coil-2 : MATLAB Function  TreatAsAtomicUnit=on
  Coil-3 : MATLAB Function  TreatAsAtomicUnit=on
  Coil-4 : MATLAB Function  TreatAsAtomicUnit=on
  Coil-5 : MATLAB Function  TreatAsAtomicUnit=on
  Out1 : Outport
  Out2 : Outport  Port=2
  Out3 : Outport  Port=3
  Out4 : Outport  Port=4
  wires:
  Add2/1 -> Out3/1
  Add1/1 -> Out2/1
  Coil-2/2(dxn_dz) -> Add1/2
  Coil-2/4(dyn_dz) -> Add3/2
  Add3/1 -> Out4/1
  Coil-3/1(dxp_dz) -> Add/3  "I_calculated"
  Coil-3/4(dyn_dz) -> Add3/3
  z_new/1 -> Coil-1/3(z_new), Coil-3/3(z_new), Coil-4/3(z_new), Coil-5/3(z_new), Coil-2/3(z_new)
  Coil-4/1(dxp_dz) -> Add/4  "I_calculated"
  Add/1 -> Out1/1
  Coil-2/1(dxp_dz) -> Add/2  "I_calculated"
  Coil-1/3(dyp_dz) -> Add2/1
  Coil-1/2(dxn_dz) -> Add1/1
  Coil-4/4(dyn_dz) -> Add3/4
  Coil-1/4(dyn_dz) -> Add3/1
  y_new/1 -> Coil-5/2(y_new), Coil-4/2(y_new), Coil-3/2(y_new), Coil-2/2(y_new), Coil-1/2(y_new)
  Coil-5/1(dxp_dz) -> Add/5  "I_calculated"
  x_new/1 -> Coil-5/1(x_new), Coil-4/1(x_new), Coil-3/1(x_new), Coil-2/1(x_new), Coil-1/1(x_new)
  Coil-1/1(dxp_dz) -> Add/1  "I_calculated"
  Coil-2/3(dyp_dz) -> Add2/2
  Coil-5/3(dyp_dz) -> Add2/5
  Coil-4/3(dyp_dz) -> Add2/4
  Coil-5/4(dyn_dz) -> Add3/5
  Coil-4/2(dxn_dz) -> Add1/4
  Coil-3/2(dxn_dz) -> Add1/3
  Coil-3/3(dyp_dz) -> Add2/3
  Coil-5/2(dxn_dz) -> Add1/5

== system I_for_8_coils_diagonal_motion/Right_Up_Coil/Left_Coil1/Outer5 Coils ==
  x_new : Inport
  y_new : Inport  Port=2
  z_new : Inport  Port=3
  Add{,1..3} (4 alike) : Sum  Inputs=+++++
  Coil-10 : MATLAB Function  TreatAsAtomicUnit=on
  Coil-6 : MATLAB Function  TreatAsAtomicUnit=on
  Coil-7 : MATLAB Function  TreatAsAtomicUnit=on
  Coil-8 : MATLAB Function  TreatAsAtomicUnit=on
  Coil-9 : MATLAB Function  TreatAsAtomicUnit=on
  Out1 : Outport
  Out2 : Outport  Port=2
  Out3 : Outport  Port=3
  Out4 : Outport  Port=4
  wires:
  Coil-10/2(dxn_dz) -> Add1/5
  Coil-8/3(dyp_dz) -> Add2/3
  Coil-8/2(dxn_dz) -> Add1/3
  Coil-9/2(dxn_dz) -> Add1/4
  Coil-10/4(dyn_dz) -> Add3/5
  Coil-9/3(dyp_dz) -> Add2/4
  Coil-10/3(dyp_dz) -> Add2/5
  Coil-7/3(dyp_dz) -> Add2/2
  Coil-6/1(dxp_dz) -> Add/1  "I_calculated"
  x_new/1 -> Coil-6/1(x_new), Coil-7/1(x_new), Coil-8/1(x_new), Coil-9/1(x_new), Coil-10/1(x_new)
  Coil-10/1(dxp_dz) -> Add/5  "I_calculated"
  y_new/1 -> Coil-6/2(y_new), Coil-7/2(y_new), Coil-8/2(y_new), Coil-9/2(y_new), Coil-10/2(y_new)
  Coil-6/4(dyn_dz) -> Add3/1
  Coil-9/4(dyn_dz) -> Add3/4
  Coil-6/2(dxn_dz) -> Add1/1
  Coil-6/3(dyp_dz) -> Add2/1
  Coil-7/1(dxp_dz) -> Add/2  "I_calculated"
  Add/1 -> Out1/1
  Coil-9/1(dxp_dz) -> Add/4  "I_calculated"
  z_new/1 -> Coil-7/3(z_new), Coil-9/3(z_new), Coil-10/3(z_new), Coil-8/3(z_new), Coil-6/3(z_new)
  Coil-8/4(dyn_dz) -> Add3/3
  Coil-8/1(dxp_dz) -> Add/3  "I_calculated"
  Add3/1 -> Out4/1
  Coil-7/4(dyn_dz) -> Add3/2
  Coil-7/2(dxn_dz) -> Add1/2
  Add1/1 -> Out2/1
  Add2/1 -> Out3/1

== system I_for_8_coils_diagonal_motion/Up_Coil/Left_Coil3/Inner 5 Coils ==
  x_new : Inport
  y_new : Inport  Port=2
  z_new : Inport  Port=3
  Add{,1..3} (4 alike) : Sum  Inputs=+++++
  Coil-1 : MATLAB Function  TreatAsAtomicUnit=on
  Coil-2 : MATLAB Function  TreatAsAtomicUnit=on
  Coil-3 : MATLAB Function  TreatAsAtomicUnit=on
  Coil-4 : MATLAB Function  TreatAsAtomicUnit=on
  Coil-5 : MATLAB Function  TreatAsAtomicUnit=on
  Out1 : Outport
  Out2 : Outport  Port=2
  Out3 : Outport  Port=3
  Out4 : Outport  Port=4
  wires:
  Coil-5/2(dxn_dz) -> Add1/5
  Coil-3/3(dyp_dz) -> Add2/3
  Coil-3/2(dxn_dz) -> Add1/3
  Coil-4/2(dxn_dz) -> Add1/4
  Coil-5/4(dyn_dz) -> Add3/5
  Coil-4/3(dyp_dz) -> Add2/4
  Coil-5/3(dyp_dz) -> Add2/5
  Coil-2/3(dyp_dz) -> Add2/2
  Coil-1/1(dxp_dz) -> Add/1  "I_calculated"
  x_new/1 -> Coil-1/1(x_new), Coil-2/1(x_new), Coil-3/1(x_new), Coil-4/1(x_new), Coil-5/1(x_new)
  Coil-5/1(dxp_dz) -> Add/5  "I_calculated"
  y_new/1 -> Coil-1/2(y_new), Coil-2/2(y_new), Coil-3/2(y_new), Coil-4/2(y_new), Coil-5/2(y_new)
  Coil-1/4(dyn_dz) -> Add3/1
  Coil-4/4(dyn_dz) -> Add3/4
  Coil-1/2(dxn_dz) -> Add1/1
  Coil-1/3(dyp_dz) -> Add2/1
  Coil-2/1(dxp_dz) -> Add/2  "I_calculated"
  Add/1 -> Out1/1
  Coil-4/1(dxp_dz) -> Add/4  "I_calculated"
  z_new/1 -> Coil-2/3(z_new), Coil-5/3(z_new), Coil-4/3(z_new), Coil-3/3(z_new), Coil-1/3(z_new)
  Coil-3/4(dyn_dz) -> Add3/3
  Coil-3/1(dxp_dz) -> Add/3  "I_calculated"
  Add3/1 -> Out4/1
  Coil-2/4(dyn_dz) -> Add3/2
  Coil-2/2(dxn_dz) -> Add1/2
  Add1/1 -> Out2/1
  Add2/1 -> Out3/1

== system I_for_8_coils_diagonal_motion/Up_Coil/Left_Coil3/Outer5 Coils ==
  x_new : Inport
  y_new : Inport  Port=2
  z_new : Inport  Port=3
  Add{,1..3} (4 alike) : Sum  Inputs=+++++
  Coil-10 : MATLAB Function  TreatAsAtomicUnit=on
  Coil-6 : MATLAB Function  TreatAsAtomicUnit=on
  Coil-7 : MATLAB Function  TreatAsAtomicUnit=on
  Coil-8 : MATLAB Function  TreatAsAtomicUnit=on
  Coil-9 : MATLAB Function  TreatAsAtomicUnit=on
  Out1 : Outport
  Out2 : Outport  Port=2
  Out3 : Outport  Port=3
  Out4 : Outport  Port=4
  wires:
  Add2/1 -> Out3/1
  Add1/1 -> Out2/1
  Coil-7/2(dxn_dz) -> Add1/2
  Coil-7/4(dyn_dz) -> Add3/2
  Add3/1 -> Out4/1
  Coil-8/1(dxp_dz) -> Add/3  "I_calculated"
  Coil-8/4(dyn_dz) -> Add3/3
  z_new/1 -> Coil-6/3(z_new), Coil-8/3(z_new), Coil-10/3(z_new), Coil-9/3(z_new), Coil-7/3(z_new)
  Coil-9/1(dxp_dz) -> Add/4  "I_calculated"
  Add/1 -> Out1/1
  Coil-7/1(dxp_dz) -> Add/2  "I_calculated"
  Coil-6/3(dyp_dz) -> Add2/1
  Coil-6/2(dxn_dz) -> Add1/1
  Coil-9/4(dyn_dz) -> Add3/4
  Coil-6/4(dyn_dz) -> Add3/1
  y_new/1 -> Coil-10/2(y_new), Coil-9/2(y_new), Coil-8/2(y_new), Coil-7/2(y_new), Coil-6/2(y_new)
  Coil-10/1(dxp_dz) -> Add/5  "I_calculated"
  x_new/1 -> Coil-10/1(x_new), Coil-9/1(x_new), Coil-8/1(x_new), Coil-7/1(x_new), Coil-6/1(x_new)
  Coil-6/1(dxp_dz) -> Add/1  "I_calculated"
  Coil-7/3(dyp_dz) -> Add2/2
  Coil-10/3(dyp_dz) -> Add2/5
  Coil-9/3(dyp_dz) -> Add2/4
  Coil-10/4(dyn_dz) -> Add3/5
  Coil-9/2(dxn_dz) -> Add1/4
  Coil-8/2(dxn_dz) -> Add1/3
  Coil-8/3(dyp_dz) -> Add2/3
  Coil-10/2(dxn_dz) -> Add1/5

== matlab function I_for_8_coils_diagonal_motion/Left_Coil/Right_Coil/Outer5 Coils/Coil-6 ==
  data: dxp_dz output; x_new input; y_new input; z_new input; dxn_dz output; dyp_dz output; dyn_dz output
function  [dxp_dz, dxn_dz, dyp_dz, dyn_dz] = current(x_new, y_new, z_new)

g = 420e-6;     %Coil spacing
m0 = 4*pi*1e-7;
radius = 3e-3;%m
height = 1e-3;%m
Magentization = 1.45; %T
vol_cy = pi*radius^2*height; % If Object is Cylinder, vol in m^3
% vol_sp = (4/3)*(pi * radius^3); % If Object is Sphere, vol in m^3

k = 0.4e-3; %additional length added to wires, to get concentric coil
%--------%--------%--------%--------%--------%--------%--------%----------
% Line along y - axis
%-%--------%--------%--------%--------%--------%--------%--------%--------
yp1_1 = -0.6e-3 - 5*k;
yp2_1 = 0.6e-3 + 5*k;
yn1_1 = -0.8e-3 - 5*k;
yn2_1 = 0.8e-3 + 5*k;
a_xp_1 = 6*g;  
a_xn_1 = -6*g;

k_yp_1 = 1/(4*pi*((a_xp_1-x_new)^2+z_new^2));
k_1yp_1 = (yp2_1-y_new)/((yp2_1-y_new)^2+(a_xp_1-x_new)^2+z_new^2)^0.5;
k_2yp_1 = (yp1_1-y_new)/((yp1_1-y_new)^2+(a_xp_1-x_new)^2+z_new^2)^0.5;

k_1yp_3 = (yp2_1-y_new)/((yp2_1-y_new)^2+(a_xp_1-x_new)^2+z_new^2)^1.5;
k_2yp_3 = (yp1_1-y_new)/((yp1_1-y_new)^2+(a_xp_1-x_new)^2+z_new^2)^1.5;

k_yn_1 = 1/(4*pi*((a_xn_1-x_new)^2+z_new^2));
k_1yn_1 = (yn2_1-y_new)/((yn2_1-y_new)^2+(a_xn_1-x_new)^2+z_new^2)^0.5;
k_2yn_1 = (yn1_1-y_new)/((yn1_1-y_new)^2+(a_xn_1-x_new)^2+z_new^2)^0.5;

k_1yn_3 = (yn2_1-y_new)/((yn2_1-y_new)^2+(a_xn_1-x_new)^2+z_new^2)^1.5;
k_2yn_3 = (yn1_1-y_new)/((yn1_1-y_new)^2+(a_xn_1-x_new)^2+z_new^2)^1.5;


hyp_z_1 = (k_yp_1) *m0;
hyp_z1_1 = (k_1yp_1 - k_2yp_1)*(-1);
hyp_z2_1 = (k_yp_1*(k_1yp_1 - k_2yp_1)*(z_new^2))*4*pi*2;
hyp_z3_1 = (k_1yp_3 - k_2yp_3)*(z_new^2);
dxp_dz = hyp_z_1*(hyp_z1_1 + hyp_z2_1 + hyp_z3_1);


hyn_z_1 = (k_yn_1)* m0*(-1);
hyn_z1_1 = (k_1yn_1 - k_2yn_1)*(-1);
hyn_z2_1 = (k_yn_1*(k_1yn_1 - k_2yn_1)*(z_new^2))*4*pi*2;
hyn_z3_1 = (k_1yn_3 - k_2yn_3)*(z_new^2);
dxn_dz = hyn_z_1*(hyn_z1_1 + hyn_z2_1 + hyn_z3_1);

%--------%--------%--------%--------%--------%--------%--------%----------
% Line along x - axis
%-%--------%--------%--------%--------%a--------%--------%--------%--------
xp1_1 = -0.8e-3 - 5*k;
xp2_1 = 0.8e-3 + 5*k;
xn1_1 = -1e-3 - 5*k;
xn2_1 = 1e-3 + 5*k;
a_yp_1 = 2.675;          %Distance of coil from (0,0)
a_yn_1 = -2.675;

k_xp_1 = 1/(4*pi*((a_yp_1-y_new)^2+z_new^2));
k_1xp_1 = (xp2_1-x_new)/((xp2_1-x_new)^2+(a_yp_1-y_new)^2+z_new^2)^0.5;
k_2xp_1 = (xp1_1-x_new)/((xp1_1-x_new)^2+(a_yp_1-y_new)^2+z_new^2)^0.5;

k_xn_1 = 1/(4*pi*((a_yn_1-y_new)^2+z_new^2));
k_1xn_1 = (xn2_1-x_new)/((xn2_1-x_new)^2+(a_yn_1-y_new)^2+z_new^2)^0.5;
k_2xn_1 = (xn1_1-x_new)/((xn1_1-x_new)^2+(a_yn_1-y_new)^2+z_new^2)^0.5;

k_1xp_3 = (xp2_1-x_new)/((xp2_1-x_new)^2+(a_yp_1-y_new)^2+z_new^2)^1.5;
k_2xp_3 = (xp1_1-x_new)/((xp1_1-x_new)^2+(a_yp_1-y_new)^2+z_new^2)^1.5;

k_1xn_3 = (xn2_1-x_new)/((xn2_1-x_new)^2+(a_yn_1-y_new)^2+z_new^2)^1.5;
k_2xn_3 = (xn1_1-x_new)/((xn1_1-x_new)^2+(a_yn_1-y_new)^2+z_new^2)^1.5;


hxp_z_1 = (k_xp_1)*m0;
hxp_z1_1 = (k_1xp_1 - k_2xp_1)*(-1);
hxp_z2_1 = (k_xp_1*(k_1xp_1 - k_2xp_1)*(z_new^2))*4*pi*2;
hxp_z3_1 = (k_1xp_3 - k_2xp_3)*(z_new^2);
dyp_dz = hxp_z_1*(hxp_z1_1 + hxp_z2_1 + hxp_z3_1);


hxn_z_1 = (k_xn_1)*m0*(-1);
hxn_z1_1 = (k_1xn_1 - k_2xn_1)*(-1);
hxn_z2_1 = (k_xn_1*(k_1xn_1 - k_2xn_1)*(z_new^2))*4*pi*2;
hxn_z3_1 = (k_1xn_3 - k_2xn_3)*(z_new^2);
dyn_dz = hxn_z_1*(hxn_z1_1 + hxn_z2_1 + hxn_z3_1);

end

== matlab function I_for_8_coils_diagonal_motion/Left_Coil/Right_Coil/Outer5 Coils/Coil-7 ==
  data: dxp_dz output; x_new input; y_new input; z_new input; dxn_dz output; dyp_dz output; dyn_dz output
function  [dxp_dz, dxn_dz, dyp_dz, dyn_dz] = current(x_new, y_new, z_new)

g = 417.14e-6;     %Coil spacing
m0 = 4*pi*1e-7;
radius = 3e-3;%m
height = 1e-3;%m
Magentization = 1.45; %T
vol_cy = pi*radius^2*height; % If Object is Cylinder, vol in m^3
% vol_sp = (4/3)*(pi * radius^3); % If Object is Sphere, vol in m^3

k = 0.4e-3; %additional length added to wires, to get concentric coil
%--------%--------%--------%--------%--------%--------%--------%----------
% Line along y - axis
%-%--------%--------%--------%--------%--------%--------%--------%--------
yp1_1 = -0.6e-3 - 6*k;
yp2_1 = 0.6e-3 + 6*k;
yn1_1 = -0.8e-3 - 6*k;
yn2_1 = 0.8e-3 + 6*k;
a_xp_1 = 7*g;  
a_xn_1 = -7*g;

k_yp_1 = 1/(4*pi*((a_xp_1-x_new)^2+z_new^2));
k_1yp_1 = (yp2_1-y_new)/((yp2_1-y_new)^2+(a_xp_1-x_new)^2+z_new^2)^0.5;
k_2yp_1 = (yp1_1-y_new)/((yp1_1-y_new)^2+(a_xp_1-x_new)^2+z_new^2)^0.5;

k_1yp_3 = (yp2_1-y_new)/((yp2_1-y_new)^2+(a_xp_1-x_new)^2+z_new^2)^1.5;
k_2yp_3 = (yp1_1-y_new)/((yp1_1-y_new)^2+(a_xp_1-x_new)^2+z_new^2)^1.5;

k_yn_1 = 1/(4*pi*((a_xn_1-x_new)^2+z_new^2));
k_1yn_1 = (yn2_1-y_new)/((yn2_1-y_new)^2+(a_xn_1-x_new)^2+z_new^2)^0.5;
k_2yn_1 = (yn1_1-y_new)/((yn1_1-y_new)^2+(a_xn_1-x_new)^2+z_new^2)^0.5;

k_1yn_3 = (yn2_1-y_new)/((yn2_1-y_new)^2+(a_xn_1-x_new)^2+z_new^2)^1.5;
k_2yn_3 = (yn1_1-y_new)/((yn1_1-y_new)^2+(a_xn_1-x_new)^2+z_new^2)^1.5;


hyp_z_1 = (k_yp_1) *m0;
hyp_z1_1 = (k_1yp_1 - k_2yp_1)*(-1);
hyp_z2_1 = (k_yp_1*(k_1yp_1 - k_2yp_1)*(z_new^2))*4*pi*2;
hyp_z3_1 = (k_1yp_3 - k_2yp_3)*(z_new^2);
dxp_dz = hyp_z_1*(hyp_z1_1 + hyp_z2_1 + hyp_z3_1);


hyn_z_1 = (k_yn_1)* m0*(-1);
hyn_z1_1 = (k_1yn_1 - k_2yn_1)*(-1);
hyn_z2_1 = (k_yn_1*(k_1yn_1 - k_2yn_1)*(z_new^2))*4*pi*2;
hyn_z3_1 = (k_1yn_3 - k_2yn_3)*(z_new^2);
dxn_dz = hyn_z_1*(hyn_z1_1 + hyn_z2_1 + hyn_z3_1);

%--------%--------%--------%--------%--------%--------%--------%----------
% Line along x - axis
%-%--------%--------%--------%--------%a--------%--------%--------%--------
xp1_1 = -0.8e-3 - 6*k;
xp2_1 = 0.8e-3 + 6*k;
xn1_1 = -1e-3 - 6*k;
xn2_1 = 1e-3 + 6*k;
a_yp_1 = 3.075;          %Distance of coil from (0,0)
a_yn_1 = -3.075;

k_xp_1 = 1/(4*pi*((a_yp_1-y_new)^2+z_new^2));
k_1xp_1 = (xp2_1-x_new)/((xp2_1-x_new)^2+(a_yp_1-y_new)^2+z_new^2)^0.5;
k_2xp_1 = (xp1_1-x_new)/((xp1_1-x_new)^2+(a_yp_1-y_new)^2+z_new^2)^0.5;

k_xn_1 = 1/(4*pi*((a_yn_1-y_new)^2+z_new^2));
k_1xn_1 = (xn2_1-x_new)/((xn2_1-x_new)^2+(a_yn_1-y_new)^2+z_new^2)^0.5;
k_2xn_1 = (xn1_1-x_new)/((xn1_1-x_new)^2+(a_yn_1-y_new)^2+z_new^2)^0.5;

k_1xp_3 = (xp2_1-x_new)/((xp2_1-x_new)^2+(a_yp_1-y_new)^2+z_new^2)^1.5;
k_2xp_3 = (xp1_1-x_new)/((xp1_1-x_new)^2+(a_yp_1-y_new)^2+z_new^2)^1.5;

k_1xn_3 = (xn2_1-x_new)/((xn2_1-x_new)^2+(a_yn_1-y_new)^2+z_new^2)^1.5;
k_2xn_3 = (xn1_1-x_new)/((xn1_1-x_new)^2+(a_yn_1-y_new)^2+z_new^2)^1.5;


hxp_z_1 = (k_xp_1)*m0;
hxp_z1_1 = (k_1xp_1 - k_2xp_1)*(-1);
hxp_z2_1 = (k_xp_1*(k_1xp_1 - k_2xp_1)*(z_new^2))*4*pi*2;
hxp_z3_1 = (k_1xp_3 - k_2xp_3)*(z_new^2);
dyp_dz = hxp_z_1*(hxp_z1_1 + hxp_z2_1 + hxp_z3_1);


hxn_z_1 = (k_xn_1)*m0*(-1);
hxn_z1_1 = (k_1xn_1 - k_2xn_1)*(-1);
hxn_z2_1 = (k_xn_1*(k_1xn_1 - k_2xn_1)*(z_new^2))*4*pi*2;
hxn_z3_1 = (k_1xn_3 - k_2xn_3)*(z_new^2);
dyn_dz = hxn_z_1*(hxn_z1_1 + hxn_z2_1 + hxn_z3_1);

end
